simulink model "CameraCalibrationModel"  (R2025b)
settings: Solver=FixedStepDiscrete  StartTime=0.0  StopTime=inf  RelTol=1e-3
model workspace (MAT data in the model file):
  patternLocation = [100 -60 0 0 0 0]
undefined symbols (not defined in the file or in its folder): Sim3dSensor
libraries: sim3dlib x4, sim3dcameralib x2, visionsinks x1
settings Model: Creator=Liam  LastModifiedBy=Liam
settings OptimizationCC: DefaultParameterBehavior=Inlined  EnhancedBackFolding=on  PassReuseOutputArgsAs=Individual arguments  ZeroExternalMemoryAtStartup=off  ZeroInternalMemoryAtStartup=off  OptimizeBlockOrder=speed  DifferentSizesBufferReuse=on  OptimizationCustomize=off  EfficientTunableParamExpr=on
settings DebuggingCC: ParameterTunabilityLossMsg=error
settings SFSimCC: MATLABDynamicMemAlloc=off
settings RTWCC: SystemTargetFile=ert.tlc  GenCodeOnly=on  TemplateMakefile=ert_default_tmf  TargetLang=C++  Description=Embedded Coder
settings CodeAppCC: ForceParamTrailComments=on  IgnoreCustomStorageClasses=off  OperatorAnnotations=on  SimulinkDataObjDesc=on  SFDataObjDesc=on  InsertBlockDesc=on
settings ERTTargetCC: RootIOFormat=Structure reference  ERTCustomFileTemplate=example_file_process.tlc  TargetLangStandard=C++11 (ISO)  GenerateSampleERTMain=on  CodeInterfacePackaging=C++ class  SubcomponentCodeInterfacePackaging=C++ class

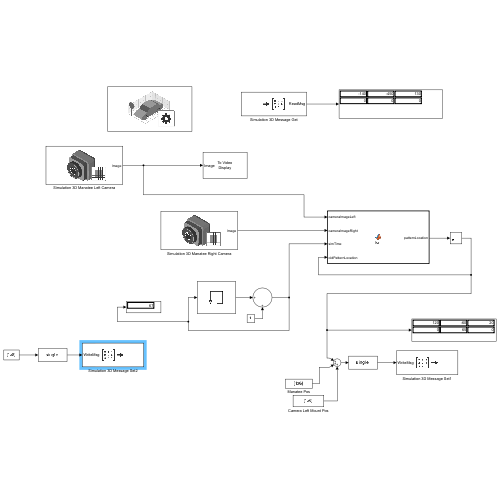
[thumbnail: Simulink's stored preview of the top-level diagram]
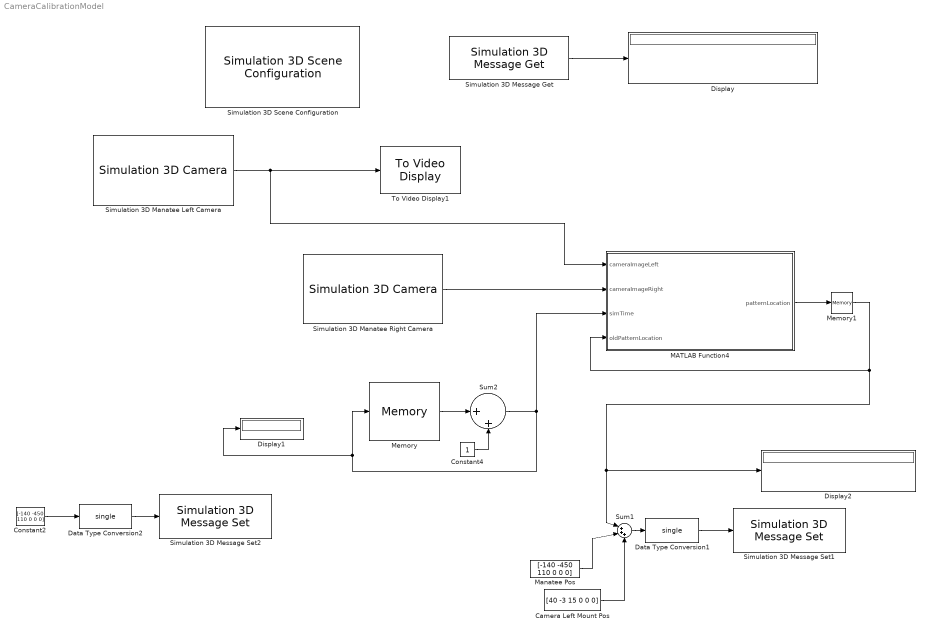
== system CameraCalibrationModel ==
  Camera Left Mount Pos : Constant  Value=[40 -3 15 0 0 0]  VectorParams1D=off  OutDataTypeStr=single
  Constant2 : Constant  Value=[-140 -450 110 0 0 0]  VectorParams1D=off  OutDataTypeStr=single
  Constant4 : Constant
  Data Type Conversion1 : DataTypeConversion  OutDataTypeStr=single  SaturateOnIntegerOverflow=off  RndMeth=Floor
  Data Type Conversion2 : DataTypeConversion  OutDataTypeStr=single  SaturateOnIntegerOverflow=off  RndMeth=Floor
  Display : Display
  Display1 : Display
  Display2 : Display
  MATLAB Function4 : MATLAB Function  TreatAsAtomicUnit=on
  Manatee Pos : Constant  Value=[-140 -450 110 0 0 0]  VectorParams1D=off  OutDataTypeStr=single
  Memory : Memory
  Memory1 : Memory  InitialCondition=[120,-60,20,0,90,0]
  Simulation 3D Manatee Left Camera : sim3dcameralib/Simulation 3D Camera  Priority=1  sensorTag=Sim3dSensor�  sensorId=1  sensorName=Sim3dSensor�  vehTagList={'Scene Origin'}  vehTag=Scene Origin  CoordinateSystem=Default  mountLoc=Origin  offsetFlag=on  tmountOffset=[40, -12.5, 15]/100  extTmount=off  rmountOffset=[0, 0, 0]  extRmount=off  FocalLength=[2.97 / 0.0028, 2.97 / 0.0028]  OpticalCenter=[960, 540]  ImageSize=[1080, 1920]  RadialDistortion=[0,0]  TangentialDistortion=[0, 0]  SensorSkew=0  VisualizeFieldOfView=off  FieldOfViewRange=61  DepthOutportEnabled=off  SemanticOutportEnabled=off  TransformOutportEnabled=off  SampleTime=-1  mountPoint=[0.4 -0.125 0.15]  mountOrientation=[0 0 0]  aMode=5  ID=1
      settings: LibrarySourceBlock=sl3dlib/Simulation 3D/Sensors/Simulation 3D Camera
  Simulation 3D Manatee Right Camera : sim3dcameralib/Simulation 3D Camera  Priority=1  sensorTag=Sim3dSensor�  sensorId=2  sensorName=Sim3dSensor�  vehTagList={'Scene Origin'}  vehTag=Scene Origin  CoordinateSystem=Default  mountLoc=Origin  offsetFlag=on  tmountOffset=[40, 12.5, 15]/100  extTmount=off  rmountOffset=[0, 0, 0]  extRmount=off  FocalLength=[2.97 / 0.0028, 2.97 / 0.0028]  OpticalCenter=[960, 540]  ImageSize=[1080, 1920]  RadialDistortion=[0,0]  TangentialDistortion=[0, 0]  SensorSkew=0  VisualizeFieldOfView=off  FieldOfViewRange=61  DepthOutportEnabled=off  SemanticOutportEnabled=off  TransformOutportEnabled=off  SampleTime=-1  mountPoint=[0.4 0.125 0.15]  mountOrientation=[0 0 0]  aMode=5  ID=2
      settings: LibrarySourceBlock=sl3dlib/Simulation 3D/Sensors/Simulation 3D Camera
  Simulation 3D Message Get : sim3dlib/Simulation 3D Message Get  Priority=1  SigName=ManateePoseGet  DataType=single  MsgSize=[1 6]  Ts=-1  aMode=0
      settings: LibrarySourceBlock=aerolibsim3d/Simulation 3D Message Get
  Simulation 3D Message Set1 : sim3dlib/Simulation 3D Message Set  Priority=-1  SigName=PatternPoseSet  Ts=-1  aMode=0
      settings: LibrarySourceBlock=aerolibsim3d/Simulation 3D Message Set
  Simulation 3D Message Set2 : sim3dlib/Simulation 3D Message Set  Priority=-1  SigName=ManateePoseSet  Ts=-1  aMode=0
      settings: LibrarySourceBlock=aerolibsim3d/Simulation 3D Message Set
  Simulation 3D Scene Configuration : sim3dlib/Simulation 3D Scene Configuration  Priority=0  ProjectFormat=Unreal Editor  SceneDesc=Straight road  ProjectName=C:\Program Files\MATLAB\R2025b\toolbox\shared\sim3d_projects\automotive_project_windows\UE\WindowsNoEditor\VehicleSimulation.exe  ScenePath=/Game/Maps/HwStrght  UEProjPath=C:\Users\Liam\OneDrive\Documents\GitHub\Vision_Sim\Unreal\UnrealProjects\SimulinkCoSimulation\EllingtonPoolSim\EllingtonPoolSim.uproject  EnableOpenDRIVE=off  vehTagList={'Custom';'Scene Origin'}  vehTag=Scene Origin  AttachedCameraRelativeTranslation=[0 0 0]  FreeCameraDefaultInitialTranslation=[-6, 0, 2]  AttachedCameraRelativeRotation=[0 0 0]  FreeCameraDefaultInitialRotation=[0, -15, 0]  ViewpointName=Custom  FreeCameraInitialTranslation=[0, 0, 0]  ViewpointTranslation=[0 0 0]  FreeCameraInitialRotation=[0, 0, 0]  ViewpointRotation=[0 0 0]  OpVisEn=off  Ts=1/60  EnableWindow=on  EnableRemoteAccess=off  EnableWeather=off  SunAzimuth=90  SunAltitude=40.0  EnableGeospatialSun=off  Latitude=0  Longitude=0  Date=2023-01-01  Time=10:30:00  GeoTimeZone=-5.0  SunDaylightSaving=off  wind=1  clouds=10  EnableVolumetricClouds=off  CloudCoverage=0  CloudAltitude=6  fog=0  rain=0  RaindropsEffect=off  SnowDensity=0  EnableGeospatial=off  TilesetSource=Earth terrain  UseTrueOrigin=off  OriginHeight=200  OriginLatitude=40.744652  OriginLongitude=-73.988864  MapStyle=Aerial  AdditionalAssetIDs=[]  UseAdvancedSunSky=off  SolarTime=11  TimeZone=-5  Day=21  Month=9  Year=2022  UseDaylightSavingTime=on  DSTStartDay=10  DSTStartMonth=3  DSTEndDay=3  DSTEndMonth=11  DSTSwitchHour=2  sensorTag=MainCamera1  sensorId=1  sensorName=MainCamera1  mountLoc=Origin  offsetFlag=off  tmountOffset=[0, 0, 0]  rmountOffset=[0, 0, 0]  HorizontalResolution=1280  VerticalResolution=720  HorizontalFOV=60  mountPoint=[0 0 0]  mountOrientation=[0 0 0]  aMode=3  ID=1  GeoTrigger=Inactive  ViewNameList={'Custom'}  ViewTranslationList={'[0 0 0]'}  ViewRotationList={'[0 0 0]'}
      settings: LibrarySourceBlock=drivingsim3d/Simulation 3D Scene Configuration
  Sum1 : Sum  Inputs=|+++
  Sum2 : Sum  Inputs=|++
  To Video Display1 : visionsinks/To Video Display  windowSizeMode=Normal  openAtMdlStart=on  fullScreen=off  videoWindowX=536805376  videoWindowY=536805376  saveWindowSize=off  videoWindowWidth=1920  videoWindowHeight=1080  inputColorFormat=RGB  inputType=Obsolete  imagePorts=One multidimensional signal  OutputDevice=On-screen video monitor  dataOrg=Column-major  isWindowOpen=off
  wires:
  Simulation 3D Manatee Left Camera/1 -> To Video Display1/1, MATLAB Function4/1(cameraImageLeft)
  Simulation 3D Message Get/1 -> Display/1
  Data Type Conversion1/1 -> Simulation 3D Message Set1/1
  Camera Left Mount Pos/1 -> Sum1/3
  Data Type Conversion2/1 -> Simulation 3D Message Set2/1
  Constant2/1 -> Data Type Conversion2/1
  Sum1/1 -> Data Type Conversion1/1
  Manatee Pos/1 -> Sum1/2
  MATLAB Function4/1(patternLocation) -> Memory1/1
  Memory/1 -> Sum2/1
  Constant4/1 -> Sum2/2
  Sum2/1 -> MATLAB Function4/3(simTime), Display1/1, Memory/1
  Memory1/1 -> Sum1/1, Display2/1, MATLAB Function4/4(oldPatternLocation)
  Simulation 3D Manatee Right Camera/1 -> MATLAB Function4/2(cameraImageRight)

== matlab function CameraCalibrationModel/MATLAB Function4 ==
  data: cameraImageLeft input; cameraImageRight input; patternLocation output; simTime input; oldPatternLocation input
function patternLocation = fcn(cameraImageLeft, cameraImageRight, simTime, oldPatternLocation)

%Pattern Boxes are each 2cm across. 20 boxes by 15 boxes. So 40cm x 30cm...
%sized grid.

coder.extrinsic('imwrite');
patternLocation = oldPatternLocation;
increment = 5;
largeIncrement = 5*increment;
time = simTime - 50;
if time <= increment * 45 && time > 0
    if mod(time, increment) == 0
        imageNameLeft = "CalibrationImages/LeftCamera/CalibrationImage" + floor(time / increment) + ".png";
        imageNameRight = "CalibrationImages/RightCamera/CalibrationImage" + floor(time / increment) + ".png";
        imwrite(cameraImageLeft, imageNameLeft);
        imwrite(cameraImageRight, imageNameRight);
        if mod(time, largeIncrement) == 0
            patternLocation(6) = 0;
            patternLocation(5) = 90;
            if patternLocation(2) == 60
                patternLocation(2) = -60;
                patternLocation(3) = patternLocation(3) - 20;
            else
                patternLocation(2) = patternLocation(2) + 60;
            end
        elseif mod(time, largeIncrement) == 1 * increment
            patternLocation(6) = 25;
            patternLocation(5) = 90;
        elseif mod(time, largeIncrement) == 2 * increment
            patternLocation(6) = -25;
            patternLocation(5) = 90;
        elseif mod(time, largeIncrement) == 3 * increment
            patternLocation(6) = 0;
            patternLocation(5) = 65;
        elseif mod(time, largeIncrement) == 4 * increment
            patternLocation(6) = 0;
            patternLocation(5) = 115;
        end
    end
end
